simulink model "QPSK"  (R2021b)
settings: Solver=ode45  StartTime=0.0  StopTime=1000  RelTol=1e-3  EnableMultiTasking=on
libraries: commdigbbndpm3 x2, commchan3 x1, commsink2 x1, commrandsrc2 x1
settings Model: Creator=Ammar  LastModifiedBy=Leon8dem1god
settings SolverCC: AlgebraicLoopSolver=TrustRegion
settings DataIOCC: LimitDataPoints=on  SaveFormat=Array  SignalLoggingSaveFormat=ModelDataLogs  ReturnWorkspaceOutputs=off
settings OptimizationCC: ExpressionDepthLimit=2147483647  LifeSpan=inf
settings DebuggingCC: UnderspecifiedInitializationDetection=Classic  MergeDetectMultiDrivingBlocksExec=none  SolverPrmCheckMsg=warning  FcnCallInpInsideContextMsg=warning  StateNameClashWarn=warning  SFUnexpectedBacktrackingDiag=warning  SFNoUnconditionalDefaultTransitionDiag=warning  SFExecutionAtInitializationDiag=none  SFMachineParentedDataDiag=warning  ArithmeticOperatorsInVariantConditions=warning
settings HardwareCC: ProdBitPerPointer=32  ProdBitPerSizeT=32  ProdBitPerPtrDiffT=32  ProdLargestAtomicFloat=None  ProdIntDivRoundTo=Undefined  ProdEndianess=Unspecified  ProdWordSize=32  ProdHWDeviceType=32-bit Generic
settings ModelReferenceCC: PropagateSignalLabelsOutOfModel=off
settings SFSimCC: SimUseLocalCustomCode=off  CustomCodeUndefinedFunction=UseInterfaceOnly
settings RTWCC: RTWUseLocalCustomCode=off
settings CodeAppCC: StateflowObjectComments=on
settings GRTTargetCC: TargetLangStandard=C89/C90 (ANSI)  CombineOutputUpdateFcns=off  GRTInterface=on
settings ConfigComp: CovMetricSettings=dw  CovSaveCumulativeToWorkspaceVar=on  CovSaveSingleToWorkspaceVar=on  CovExternalEMLEnable=off

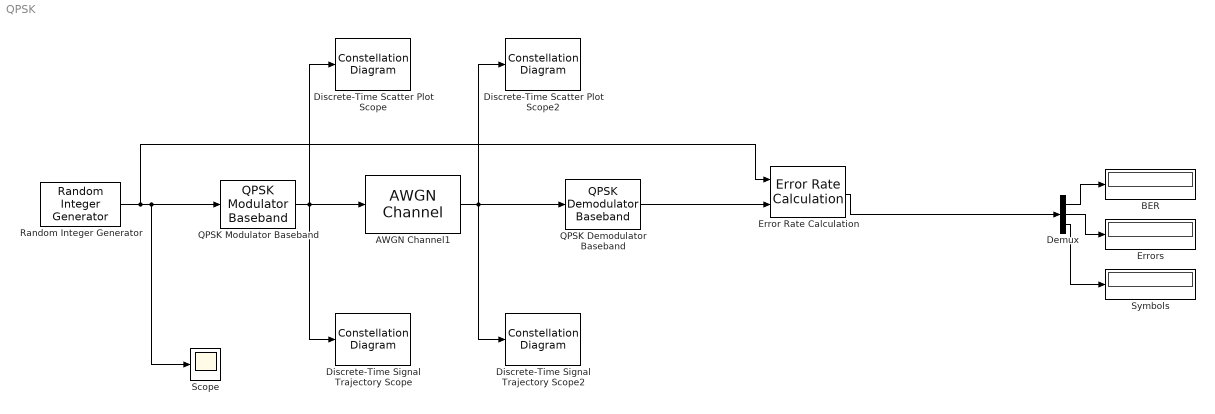
== system QPSK ==
  AWGN Channel1 : commchan3/AWGN Channel  InputProcessing=Columns as channels (frame based)  seed=67  noiseMode="Signal to noise ratio  (Eb/No)"  EbNodB=10  EsNodB=6  SNRdB=3  bitsPerSym=2  Ps=1  Tsym=1/10000  variance=1
  BER : Display
  Demux : Demux  Outputs=3
  Discrete-Time Scatter Plot Scope : ConstellationDiagram  Tag=ScatterPlot
  Discrete-Time Scatter Plot Scope2 : ConstellationDiagram  Tag=ScatterPlot
  Discrete-Time Signal Trajectory Scope : ConstellationDiagram  Tag=SignalTrajectory
  Discrete-Time Signal Trajectory Scope2 : ConstellationDiagram  Tag=SignalTrajectory
  Error Rate Calculation : commsink2/Error Rate Calculation  N=0  st_delay=0  cp_mode=Entire frame  subframe=[]  PMode=Port  WsName=ErrorVec  RsMode2=off  stop=off  numErr=100  maxBits=1e6
  Errors : Display
  QPSK Demodulator Baseband : commdigbbndpm3/QPSK Demodulator Baseband  OutType=Integer  DecType=Hard decision  VarSource=Dialog  Variance=1  Dec=Gray  Ph=pi/4  outDtype1=Inherit via internal rule  outDtype2=Inherit via internal rule  derotateFactorWordLen=16  derotateFactorDataTypeStr=Inherit: Same word length as input  derotateFactorLastDataTypeStr=Inherit: Same word length as input
  QPSK Modulator Baseband : commdigbbndpm3/QPSK Modulator Baseband  InType=Integer  Enc=Gray  Ph=pi/4  outDtype=double  outWordLen=16  outUDDataType=sfix(16)  outFracLenMode=Best precision  outFracLen=15  outDataTypeStr=double  outLastDataTypeStr=double
  Random Integer Generator : commrandsrc2/Random Integer Generator  mul=4  seed=35  Ts=1/10000  frameBased=off  sampPerFrame=1  orient=off  outDataType=double
      settings: SourceProductBaseCode=CM
  Scope : Scope
  Symbols : Display
  wires:
  Random Integer Generator/1 -> Scope/1, QPSK Modulator Baseband/1, Error Rate Calculation/1
  Demux/1 -> BER/1
  Demux/2 -> Errors/1
  Demux/3 -> Symbols/1
  Error Rate Calculation/1 -> Demux/1
  QPSK Modulator Baseband/1 -> Discrete-Time Signal Trajectory Scope/1, Discrete-Time Scatter Plot Scope/1, AWGN Channel1/1
  AWGN Channel1/1 -> Discrete-Time Signal Trajectory Scope2/1, Discrete-Time Scatter Plot Scope2/1, QPSK Demodulator Baseband/1
  QPSK Demodulator Baseband/1 -> Error Rate Calculation/2
